simulink model "Lab42"  (R2020b)
settings: Solver=VariableStepAuto  StartTime=0.0  StopTime=10.0  RelTol=1e-3
settings Model: Creator=evpet  LastModifiedBy=evpet

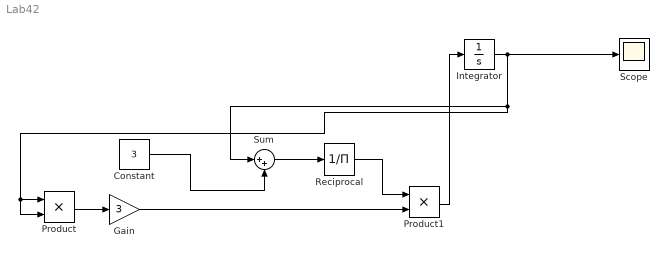
== system Lab42 ==
  Constant : Constant  Value=3
  Gain : Gain  Gain=3
  Integrator : Integrator  InitialCondition=10
  Product : Product
  Product1 : Product
  Reciprocal : Product  Inputs=/
  Scope : Scope
  Sum : Sum  Inputs=|++
  wires:
  Integrator/1 -> Sum/1, Product/1, Product/2, Scope/1
  Product/1 -> Gain/1
  Gain/1 -> Product1/2
  Constant/1 -> Sum/2
  Sum/1 -> Reciprocal/1
  Reciprocal/1 -> Product1/1
  Product1/1 -> Integrator/1
